simulink model "surazR2012bslx"  (R2018a)
settings: Solver=ode45  StartTime=0.0  StopTime=10  MaxStep=0.0001  RelTol=1e-8  EnableMultiTasking=on
settings Model: Creator=user  LastModifiedBy=user
settings DataIOCC: LimitDataPoints=on  SaveFormat=StructureWithTime  SaveOutput=off  SaveTime=off
settings OptimizationCC: ExpressionDepthLimit=2147483647  LifeSpan=1
settings DebuggingCC: UnderspecifiedInitializationDetection=Classic  MergeDetectMultiDrivingBlocksExec=none  FcnCallInpInsideContextMsg=warning  StateNameClashWarn=warning  SFUnexpectedBacktrackingDiag=warning  SFNoUnconditionalDefaultTransitionDiag=warning  SFExecutionAtInitializationDiag=none
settings HardwareCC: ProdBitPerSizeT=32  ProdBitPerPtrDiffT=32  ProdWordSize=32  ProdHWDeviceType=Specified
settings CodeAppCC: StateflowObjectComments=on
settings GRTTargetCC: TargetLangStandard=C89/C90 (ANSI)  GeneratePreprocessorConditionals=Disable all  CombineOutputUpdateFcns=off  GRTInterface=on

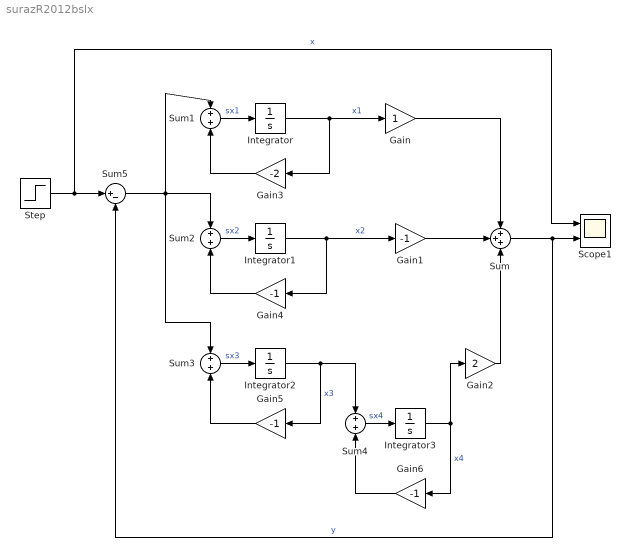
== system surazR2012bslx ==
  Gain : Gain
  Gain{1,4..6} (4 alike) : Gain  Gain=-1
  Gain2 : Gain  Gain=2
  Gain3 : Gain  Gain=-2
  Integrator{,1..3} (4 alike) : Integrator
  Scope1 : Scope  NumInputPorts=2
  Step : Step  Description=skok jednostkowy  SampleTime=0
  Sum : Sum  Inputs=3
  Sum{1..4} (4 alike) : Sum  Inputs=2
  Sum5 : Sum  Inputs=|+-
  wires:
  Sum/1 -> Sum5/2, Scope1/2  "y"
  Sum1/1 -> Integrator/1  "sx1"
  Integrator/1 -> Gain3/1, Gain/1  "x1"
  Gain3/1 -> Sum1/2
  Gain4/1 -> Sum2/2
  Sum2/1 -> Integrator1/1  "sx2"
  Integrator1/1 -> Gain4/1, Gain1/1  "x2"
  Sum3/1 -> Integrator2/1  "sx3"
  Gain5/1 -> Sum3/2
  Gain1/1 -> Sum/2
  Gain/1 -> Sum/1
  Gain2/1 -> Sum/3
  Sum4/1 -> Integrator3/1  "sx4"
  Integrator2/1 -> Gain5/1, Sum4/1  "x3"
  Integrator3/1 -> Gain2/1, Gain6/1  "x4"
  Gain6/1 -> Sum4/2
  Step/1 -> Scope1/1, Sum5/1  "x"
  Sum5/1 -> Sum3/1, Sum2/1, Sum1/1
